simulink model "CryoDetHcd"  (R2016b)
settings: Solver=ode45  StartTime=0.0  StopTime=1e-3  RelTol=1e-3
PreLoadFcn:
  | setup_hcd
values from neighbouring files (symbols this model uses):
  A = sqrt(0.5*erfc(x))    [setup_hcd.m]
  etaRomData = zeros(1,128)    [setup_hcd.m]
  Fadc = 614e6    (= 614000000)    [setup_hcd.m]
  freqRomData = zeros(1,128)    [setup_hcd.m]
  freqRomData1 = zeros(1,128)    [setup_hcd.m]
  freqRomData2 = zeros(1,128)    [setup_hcd.m]
  freqRomData3 = zeros(1,128)    [setup_hcd.m]
undefined symbols (not defined in the file or in its folder): AXI4, B, C, D, j, Lite
libraries: xbsIndex_r4 x2151, CryoDetLibCMB x28, hdlsllib x8, dspsigops x2, simulink x1
(part 4 of 17)

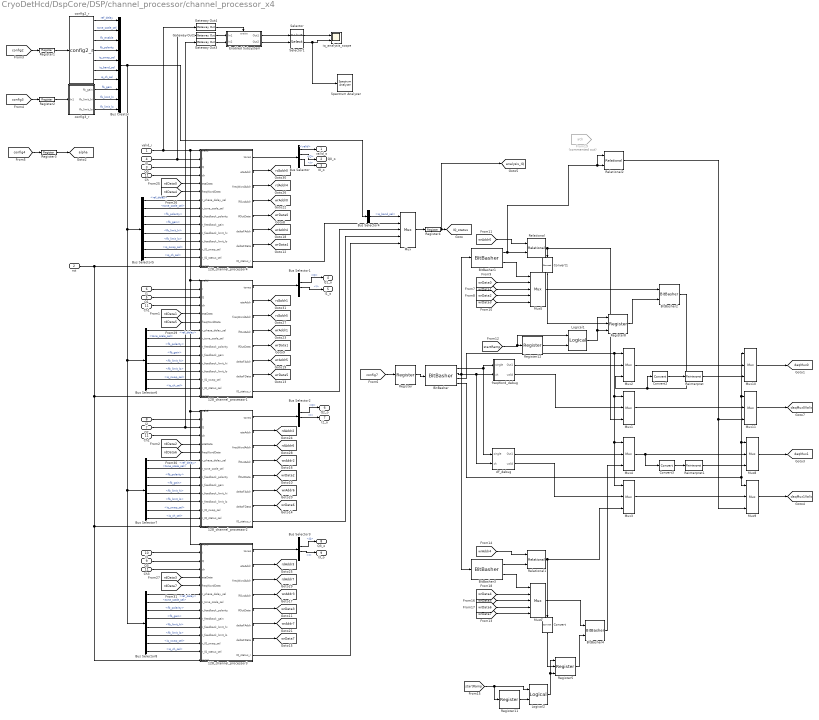
== system CryoDetHcd/DspCore/DSP/channel_processor/channel_processor_x4 ==
  valid_i : Inport
  rst : Inport  Port=2
  Q0 : Inport  Port=3
  I0 : Inport  Port=4
  Q1 : Inport  Port=5
  I1 : Inport  Port=6
  Q2 : Inport  Port=7
  I2 : Inport  Port=8
  Q3 : Inport  Port=9
  I3 : Inport  Port=10
  Ch : Inport  Port=11
  128_channel_processor1 : Subsystem  AncestorBlock=CryoDetLibCMB/128_channel_processor
  128_channel_processor2 : Subsystem  AncestorBlock=CryoDetLibCMB/128_channel_processor
  128_channel_processor3 : Subsystem  AncestorBlock=CryoDetLibCMB/128_channel_processor
  128_channel_processor4 : Subsystem  AncestorBlock=CryoDetLibCMB/128_channel_processor
  BitBasher : xbsIndex_r4/BitBasher  bitexpr=|  display_expr=off  sr_1=single_channel  arith_type1=Unsigned  bin_pt1=0  sr_2=channel_select  arith_type2=Unsigned  bin_pt2=0  sr_3=mode2  arith_type3=Unsigned  bin_pt3=0  sr_4=mode3  arith_type4=Unsigned  bin_pt4=0  dbl_ovrd=off  block_type=bitbasher
      | single_channel = {in[0]}
      | channel_select = {in[9:1]}
      | mode2 = {in[10]}
      | mode3 = {in[11]}
  BitBasher1 : xbsIndex_r4/BitBasher  bitexpr=|  display_expr=off  sr_1=ch  arith_type1=Unsigned  bin_pt1=0  sr_2=stream  arith_type2=Unsigned  bin_pt2=0  sr_3=mode2  arith_type3=Unsigned  bin_pt3=0  sr_4=4  arith_type4=Unsigned  bin_pt4=0  dbl_ovrd=off  block_type=bitbasher
      | ch = {in[6:0]}
      | stream = {in[8:7]}
  BitBasher2 : xbsIndex_r4/BitBasher  bitexpr=out = {ramp, 7'b0, in[23:0]}  display_expr=off  sr_1=out  arith_type1=Unsigned  bin_pt1=0  sr_2=channel_select  arith_type2=Unsigned  bin_pt2=0  sr_3=mode2  arith_type3=Unsigned  bin_pt3=0  sr_4=4  arith_type4=Unsigned  bin_pt4=0  dbl_ovrd=off  block_type=bitbasher
  BitBasher3 : xbsIndex_r4/BitBasher  bitexpr=|  display_expr=off  sr_1=ch  arith_type1=Unsigned  bin_pt1=0  sr_2=stream  arith_type2=Unsigned  bin_pt2=0  sr_3=mode2  arith_type3=Unsigned  bin_pt3=0  sr_4=4  arith_type4=Unsigned  bin_pt4=0  dbl_ovrd=off  block_type=bitbasher
      | ch = {in[6:0]}
      | stream = {in[8:7]}
  BitBasher4 : xbsIndex_r4/BitBasher  bitexpr=out = {ramp, 7'b0, in[23:0]}  display_expr=off  sr_1=out  arith_type1=Unsigned  bin_pt1=0  sr_2=channel_select  arith_type2=Unsigned  bin_pt2=0  sr_3=mode2  arith_type3=Unsigned  bin_pt3=0  sr_4=4  arith_type4=Unsigned  bin_pt4=0  dbl_ovrd=off  block_type=bitbasher
  Bus Creator : BusCreator  Inputs=10
  Bus Selector{,1..3} (4 alike) : BusSelector  OutputSignals=valid,Q,I,ch
  Bus Selector4 : BusSelector  OutputSignals=iq_band_sel
  Bus Selector{5..8} (4 alike) : BusSelector  OutputSignals=ref_delay,tone_scale_sel,fb_polarity,fb_gain,fb_limit_hi,fb_limit_lo,iq_swap_sel,iq_ch_sel
  Ch1 : InportShadow  Port=11
  Ch2 : InportShadow  Port=11
  Ch3 : InportShadow  Port=11
  Convert : xbsIndex_r4/Convert  gui_display_data_type=Boolean  arith_type=Boolean  n_bits=16  bin_pt=14  float_type=Single  exp_bits=8  fraction_bits=24  quantization=Truncate  overflow=Wrap  en=off  latency=0  pipeline=off  dbl_ovrd=off  block_type=convert
  Convert1 : xbsIndex_r4/Convert  gui_display_data_type=Boolean  arith_type=Boolean  n_bits=16  bin_pt=14  float_type=Single  exp_bits=8  fraction_bits=24  quantization=Truncate  overflow=Wrap  en=off  latency=0  pipeline=off  dbl_ovrd=off  block_type=convert
  Convert2 : xbsIndex_r4/Convert  gui_display_data_type=Fixed-point  arith_type="Signed  (2's comp)"  n_bits=32  bin_pt=32  float_type=Single  exp_bits=8  fraction_bits=24  quantization=Truncate  overflow=Wrap  en=off  latency=1  pipeline=off  dbl_ovrd=off  block_type=convert
  Convert3 : xbsIndex_r4/Convert  gui_display_data_type=Fixed-point  arith_type="Signed  (2's comp)"  n_bits=32  bin_pt=32  float_type=Single  exp_bits=8  fraction_bits=24  quantization=Truncate  overflow=Wrap  en=off  latency=1  pipeline=off  dbl_ovrd=off  block_type=convert
  Enabled Subsystem : Subsystem  TreatAsAtomicUnit=on
  From19 : From  Commented=on  GotoTag=aCh
  Gateway Out1 : xbsIndex_r4/Gateway Out  inherit_from_input=on  hdl_port=off  rows=1  columns=1  UseAsDAC=off  DACChannel='1'  interface=None  automatic_assignment=on  address_offset=hex2dec('00')  intf_name=''  intf_description=''  timing_constraint=None  locs_specified=off  LOCs={}  io_standard={}  block_type=gatewayout
  Gateway Out3 : xbsIndex_r4/Gateway Out  inherit_from_input=on  hdl_port=off  rows=1  columns=1  UseAsDAC=off  DACChannel='1'  interface=None  automatic_assignment=on  address_offset=hex2dec('00')  intf_name=''  intf_description=''  timing_constraint=None  locs_specified=off  LOCs={}  io_standard={}  block_type=gatewayout
  Gateway Out4 : xbsIndex_r4/Gateway Out  inherit_from_input=on  hdl_port=off  rows=1  columns=1  UseAsDAC=off  DACChannel='1'  interface=None  automatic_assignment=on  address_offset=hex2dec('00')  intf_name=''  intf_description=''  timing_constraint=None  locs_specified=off  LOCs={}  io_standard={}  block_type=gatewayout
  Logical1 : xbsIndex_r4/Logical  logical_function=OR  inputs=2  en=off  latency=0  precision=User Defined  arith_type=Boolean  n_bits=16  bin_pt=0  align_bp=on  dbl_ovrd=off  block_type=logical
  Logical2 : xbsIndex_r4/Logical  logical_function=OR  inputs=2  en=off  latency=0  precision=User Defined  arith_type=Boolean  n_bits=16  bin_pt=0  align_bp=on  dbl_ovrd=off  block_type=logical
  Mux : xbsIndex_r4/Mux  inputs=4  en=off  latency=1  precision=Full  arith_type=Unsigned  n_bits=16  bin_pt=14  quantization=Truncate  overflow=Wrap  dbl_ovrd=off  block_type=mux
  Mux{1..4,8..11} (8 alike) : xbsIndex_r4/Mux  inputs=2  en=off  latency=1  precision=Full  arith_type=Unsigned  n_bits=16  bin_pt=14  quantization=Truncate  overflow=Wrap  dbl_ovrd=off  block_type=mux
  Mux5 : xbsIndex_r4/Mux  inputs=4  en=off  latency=1  precision=Full  arith_type=Unsigned  n_bits=16  bin_pt=14  quantization=Truncate  overflow=Wrap  dbl_ovrd=off  block_type=mux
  Mux6 : xbsIndex_r4/Mux  inputs=4  en=off  latency=1  precision=Full  arith_type=Unsigned  n_bits=16  bin_pt=14  quantization=Truncate  overflow=Wrap  dbl_ovrd=off  block_type=mux
  Register{,1..4,11..12} (7 alike) : xbsIndex_r4/Register  init=0  rst=off  en=off  dbl_ovrd=off  block_type=register
  Register5 : xbsIndex_r4/Register  init=0  rst=on  en=on  dbl_ovrd=off  block_type=register
  Register8 : xbsIndex_r4/Register  init=0  rst=on  en=on  dbl_ovrd=off  block_type=register
  Reinterpret : xbsIndex_r4/Reinterpret  force_arith_type=on  arith_type=Unsigned  force_bin_pt=on  bin_pt=0  block_type=reinterpret
  Reinterpret1 : xbsIndex_r4/Reinterpret  force_arith_type=on  arith_type=Unsigned  force_bin_pt=on  bin_pt=0  block_type=reinterpret
  Relational : xbsIndex_r4/Relational  mode=a=b  op_type=Ufix  en=off  latency=1  dbl_ovrd=off  block_type=relational
  Relational1 : xbsIndex_r4/Relational  mode=a=b  op_type=Ufix  en=off  latency=1  dbl_ovrd=off  block_type=relational
  Relational2 : xbsIndex_r4/Relational  mode=a=b  op_type=Ufix  en=off  latency=1  dbl_ovrd=off  block_type=relational
  Selector : Selector  InputPortWidth=8  IndexOptions=Index vector (dialog)  Indices=[1]  OutputSizes=1
  Selector1 : Selector  InputPortWidth=8  IndexOptions=Index vector (dialog)  Indices=[1]  OutputSizes=1
  Spectrum Analyzer : SpectrumAnalyzer
  config2_r : CryoDetLibCMB/config2_r
  config3_r : Subsystem  AncestorBlock=CryoDetLibCMB/config3_r
  dF_debug : Subsystem
  freqWord_debug : Subsystem
  iq_analysis_scope : Scope  NumInputPorts=2
  valid_o : Outport
  Q0_o : Outport  Port=2
  I0_o : Outport  Port=3
  Q1_o : Outport  Port=4
  I1_o : Outport  Port=5
  Q2_o : Outport  Port=6
  I2_o : Outport  Port=7
  Q3_o : Outport  Port=8
  I3_o : Outport  Port=9
  tag scope: IQ_status=global, alpha=global, analysis_IQ=global, daqMux0=global, daqMux0Valid=global, daqMux1=global, daqMux1Valid=global, rdAddr0=global, rdAddr1=global, rdAddr2=global, rdAddr3=global, rdAddr4=global, rdAddr5=global, rdAddr6=global, rdAddr7=global, wrAddr0=global, wrAddr1=global, wrAddr2=global, wrAddr3=global, wrAddr4=global, wrAddr5=global, wrAddr6=global, wrAddr7=global, wrData0=global, wrData1=global, wrData2=global, wrData3=global, wrData4=global, wrData5=global, wrData6=global, wrData7=global
  wires:
  128_channel_processor3/8(IQ_status_r) -> Mux/5
  128_channel_processor2/8(IQ_status_r) -> Mux/4
  128_channel_processor1/8(IQ_status_r) -> Mux/3
  128_channel_processor4/8(IQ_status_r) -> Mux/2
  Register4/1 -> [analysis_IQ], [IQ_status]
  Mux/1 -> Register4/1
  Bus Selector/1 -> valid_o/1  "<valid>"
  [rdData3] -> 128_channel_processor3/5(etaData)
  [rdData7] -> 128_channel_processor3/6(freqWordData)
  [rdData6] -> 128_channel_processor2/6(freqWordData)
  [rdData2] -> 128_channel_processor2/5(etaData)
  [rdData5] -> 128_channel_processor1/6(freqWordData)
  [rdData1] -> 128_channel_processor1/5(etaData)
  128_channel_processor2/2(etaAddr) -> [rdAddr2]
  128_channel_processor2/3(freqWordAddr) -> [rdAddr6]
  128_channel_processor3/2(etaAddr) -> [rdAddr3]
  128_channel_processor3/3(freqWordAddr) -> [rdAddr7]
  128_channel_processor1/2(etaAddr) -> [rdAddr1]
  128_channel_processor1/3(freqWordAddr) -> [rdAddr5]
  128_channel_processor3/7(deltaFData) -> [wrData7]
  128_channel_processor3/6(deltaFAddr) -> [wrAddr7]
  128_channel_processor3/5(lfOutData) -> [wrData3]
  128_channel_processor3/4(lfOutAddr) -> [wrAddr3]
  128_channel_processor2/7(deltaFData) -> [wrData6]
  128_channel_processor2/6(deltaFAddr) -> [wrAddr6]
  128_channel_processor2/5(lfOutData) -> [wrData2]
  128_channel_processor2/4(lfOutAddr) -> [wrAddr2]
  128_channel_processor1/4(lfOutAddr) -> [wrAddr1]
  128_channel_processor1/5(lfOutData) -> [wrData1]
  128_channel_processor1/6(deltaFAddr) -> [wrAddr5]
  128_channel_processor1/7(deltaFData) -> [wrData5]
  Q1/1 -> 128_channel_processor1/3(Q)
  I1/1 -> 128_channel_processor1/2(I)
  I2/1 -> 128_channel_processor2/2(I)
  I3/1 -> 128_channel_processor3/2(I)
  Q3/1 -> 128_channel_processor3/3(Q)
  Bus Selector3/3 -> I3_o/1  "<I>"
  Bus Selector3/2 -> Q3_o/1  "<Q>"
  Bus Selector2/3 -> I2_o/1  "<I>"
  Bus Selector2/2 -> Q2_o/1  "<Q>"
  Bus Selector1/3 -> I1_o/1  "<I>"
  Bus Selector1/2 -> Q1_o/1  "<Q>"
  128_channel_processor3/1(tones) -> Bus Selector3/1
  128_channel_processor2/1(tones) -> Bus Selector2/1
  128_channel_processor1/1(tones) -> Bus Selector1/1
  Bus Selector/3 -> I0_o/1  "<I>"
  Bus Selector/2 -> Q0_o/1  "<Q>"
  128_channel_processor4/1(tones) -> Bus Selector/1
  Ch/1 -> 128_channel_processor4/4(ch)
  [rdData4] -> 128_channel_processor4/6(freqWordData)
  [rdData0] -> 128_channel_processor4/5(etaData)
  128_channel_processor4/7(deltaFData) -> [wrData4]
  128_channel_processor4/5(lfOutData) -> [wrData0]
  128_channel_processor4/4(lfOutAddr) -> [wrAddr0]
  128_channel_processor4/6(deltaFAddr) -> [wrAddr4]
  128_channel_processor4/2(etaAddr) -> [rdAddr0]
  128_channel_processor4/3(freqWordAddr) -> [rdAddr4]
  [config2] -> Register1/1
  [config3] -> Register2/1
  Register2/1 -> config3_r/1(In1)
  Register1/1 -> config2_r/1
  config2_r/5 -> Bus Creator/5  "iq_swap_sel"
  config2_r/7 -> Bus Creator/7  "iq_ch_sel"
  config2_r/6 -> Bus Creator/6  "iq_band_sel"
  config2_r/1 -> Bus Creator/1  "ref_delay"
  config2_r/2 -> Bus Creator/2  "tone_scale_sel"
  config2_r/3 -> Bus Creator/3  "fb_enable"
  config2_r/4 -> Bus Creator/4  "fb_polarity"
  config3_r/1(fb_gain) -> Bus Creator/8  "fb_gain"
  config3_r/2(fb_limit_hi) -> Bus Creator/9  "fb_limit_hi"
  Bus Selector4/1 -> Mux/1  "<iq_band_sel>"
  Bus Creator/1 -> Bus Selector4/1, Bus Selector6/1, Bus Selector8/1, Bus Selector7/1, Bus Selector5/1
  Ch1/1 -> 128_channel_processor1/4(ch)
  Ch2/1 -> 128_channel_processor2/4(ch)
  Ch3/1 -> 128_channel_processor3/4(ch)
  config3_r/3(fb_limit_lo) -> Bus Creator/10  "fb_limit_lo"
  Bus Selector5/2 -> 128_channel_processor4/8(r_tone_scale_sel)  "<tone_scale_sel>"
  Bus Selector5/3 -> 128_channel_processor4/9(r_feedback_polarity)  "<fb_polarity>"
  Bus Selector5/1 -> 128_channel_processor4/7(r_phase_delay_sel)  "<ref_delay>"
  Bus Selector5/4 -> 128_channel_processor4/10(r_feedback_gain)  "<fb_gain>"
  Bus Selector5/5 -> 128_channel_processor4/11(r_feedback_limit_hi)  "<fb_limit_hi>"
  Bus Selector5/6 -> 128_channel_processor4/12(r_feedback_limit_lo)  "<fb_limit_lo>"
  Bus Selector5/7 -> 128_channel_processor4/13(r_IQ_swap_sel)  "<iq_swap_sel>"
  Bus Selector5/8 -> 128_channel_processor4/14(r_IQ_status_sel)  "<iq_ch_sel>"
  Bus Selector6/7 -> 128_channel_processor1/13(r_IQ_swap_sel)  "<iq_swap_sel>"
  Bus Selector6/8 -> 128_channel_processor1/14(r_IQ_status_sel)  "<iq_ch_sel>"
  Bus Selector6/1 -> 128_channel_processor1/7(r_phase_delay_sel)  "<ref_delay>"
  Bus Selector6/4 -> 128_channel_processor1/10(r_feedback_gain)  "<fb_gain>"
  Bus Selector6/5 -> 128_channel_processor1/11(r_feedback_limit_hi)  "<fb_limit_hi>"
  Bus Selector6/6 -> 128_channel_processor1/12(r_feedback_limit_lo)  "<fb_limit_lo>"
  Bus Selector6/3 -> 128_channel_processor1/9(r_feedback_polarity)  "<fb_polarity>"
  Bus Selector6/2 -> 128_channel_processor1/8(r_tone_scale_sel)  "<tone_scale_sel>"
  Bus Selector7/6 -> 128_channel_processor2/12(r_feedback_limit_lo)  "<fb_limit_lo>"
  Bus Selector7/1 -> 128_channel_processor2/7(r_phase_delay_sel)  "<ref_delay>"
  Bus Selector7/5 -> 128_channel_processor2/11(r_feedback_limit_hi)  "<fb_limit_hi>"
  Bus Selector7/2 -> 128_channel_processor2/8(r_tone_scale_sel)  "<tone_scale_sel>"
  Bus Selector7/7 -> 128_channel_processor2/13(r_IQ_swap_sel)  "<iq_swap_sel>"
  Bus Selector7/3 -> 128_channel_processor2/9(r_feedback_polarity)  "<fb_polarity>"
  Bus Selector7/4 -> 128_channel_processor2/10(r_feedback_gain)  "<fb_gain>"
  Bus Selector7/8 -> 128_channel_processor2/14(r_IQ_status_sel)  "<iq_ch_sel>"
  rst/1 -> 128_channel_processor4/15(reset), 128_channel_processor1/15(reset), 128_channel_processor3/15(reset), 128_channel_processor2/15(reset)
  Bus Selector8/8 -> 128_channel_processor3/14(r_IQ_status_sel)  "<iq_ch_sel>"
  Bus Selector8/4 -> 128_channel_processor3/10(r_feedback_gain)  "<fb_gain>"
  Bus Selector8/2 -> 128_channel_processor3/8(r_tone_scale_sel)  "<tone_scale_sel>"
  Bus Selector8/3 -> 128_channel_processor3/9(r_feedback_polarity)  "<fb_polarity>"
  Bus Selector8/1 -> 128_channel_processor3/7(r_phase_delay_sel)  "<ref_delay>"
  Bus Selector8/5 -> 128_channel_processor3/11(r_feedback_limit_hi)  "<fb_limit_hi>"
  Bus Selector8/6 -> 128_channel_processor3/12(r_feedback_limit_lo)  "<fb_limit_lo>"
  Bus Selector8/7 -> 128_channel_processor3/13(r_IQ_swap_sel)  "<iq_swap_sel>"
  [config4] -> Register3/1
  Register3/1 -> [alpha]
  I0/1 -> Gateway Out1/1, 128_channel_processor4/2(I)
  Q0/1 -> 128_channel_processor4/3(Q)
  valid_i/1 -> Gateway Out4/1, 128_channel_processor4/1(valid), 128_channel_processor1/1(valid), 128_channel_processor3/1(valid), 128_channel_processor2/1(valid)
  Enabled Subsystem/2(Out2) -> Selector1/1
  Enabled Subsystem/1(Out1) -> Selector/1
  Selector1/1 -> Spectrum Analyzer/1, iq_analysis_scope/2
  Selector/1 -> iq_analysis_scope/1
  Gateway Out1/1 -> Enabled Subsystem/1(In1)
  Gateway Out3/1 -> Enabled Subsystem/2(In2)
  Gateway Out4/1 -> Enabled Subsystem/Enable
  Q2/1 -> 128_channel_processor2/3(Q), Gateway Out3/1
  [config7] -> Register/1
  Register/1 -> BitBasher/1
  BitBasher/1 -> freqWord_debug/1(single), dF_debug/1(single)
  BitBasher/2 -> BitBasher3/1, BitBasher1/1, dF_debug/2(ch), freqWord_debug/2(ch)
  freqWord_debug/1(Out1) -> Mux2/2
  freqWord_debug/2(valid) -> Mux1/2
  BitBasher/3 -> Mux4/1, Mux3/1, Mux1/1, Mux2/1
  dF_debug/1(Out1) -> Mux4/2
  dF_debug/2(valid) -> Mux3/2
  BitBasher1/2 -> Mux5/1
  [wrData0] -> Mux5/2
  [wrData1] -> Mux5/3
  [wrData3] -> Mux5/5
  [wrData2] -> Mux5/4
  [wrAddr0] -> Relational/1
  BitBasher3/2 -> Mux6/1
  [wrData4] -> Mux6/2
  [wrData5] -> Mux6/3
  [wrData7] -> Mux6/5
  [wrData6] -> Mux6/4
  BitBasher3/1 -> Relational1/2
  [wrAddr4] -> Relational1/1
  BitBasher4/1 -> Mux4/3
  Mux6/1 -> BitBasher4/1
  Relational1/1 -> Mux3/3, Convert/1
  Mux5/1 -> BitBasher2/1
  Relational/1 -> Mux1/3, Convert1/1
  [startRamp] -> Logical1/1, Register12/1
  [startRamp] -> Register11/1, Logical2/1
  Convert/1 -> Register5/2
  Convert1/1 -> Register8/2
  Register8/1 -> BitBasher2/2
  Register12/1 -> Logical1/2
  Logical1/1 -> Register8/1, Register8/3
  Register11/1 -> Logical2/2
  Logical2/1 -> Register5/1, Register5/3
  Register5/1 -> BitBasher4/2
  BitBasher2/1 -> Convert2/1, Mux2/3
  Mux4/1 -> Convert3/1, Mux8/2
  Mux8/1 -> [daqMux1]
  Mux3/1 -> Mux9/2
  Mux9/1 -> [daqMux1Valid]
  Mux1/1 -> Mux11/2
  Mux11/1 -> [daqMux0Valid]
  Mux2/1 -> Mux10/2
  Mux10/1 -> [daqMux0]
  Convert3/1 -> Reinterpret1/1
  Convert2/1 -> Reinterpret/1
  Relational2/1 -> Mux9/3, Mux11/3
  BitBasher/4 -> Mux9/1, Mux11/1, Mux10/1, Mux8/1
  Reinterpret/1 -> Mux10/3
  Reinterpret1/1 -> Mux8/3
  BitBasher1/1 -> Relational2/1, Relational2/2, Relational/2

== system CryoDetHcd/DspCore/DSP/Synthesis_pipelined/Synthesis/Combine ==
  valid : Inport
  im0 : Inport  Port=2
  re0 : Inport  Port=3
  im1 : Inport  Port=4
  re1 : Inport  Port=5
  Add2 : Sum
  AddSub{,1..3} (4 alike) : xbsIndex_r4/AddSub  mode=Subtraction  use_carryin=off  use_carryout=off  en=off  latency=2  precision=User Defined  arith_type="Signed  (2's comp)"  n_bits=16  bin_pt=15  quantization=Truncate  overflow=Saturate  use_behavioral_HDL=on  hw_selection=Fabric  pipelined=off  dbl_ovrd=off  block_type=addsub
  BitBasher1 : xbsIndex_r4/BitBasher  bitexpr=|  display_expr=off  sr_1=hi  arith_type1="Signed  (2's comp)"  bin_pt1=15  sr_2=lo  arith_type2="Signed  (2's comp)"  bin_pt2=15  sr_3=hi  arith_type3=Unsigned  bin_pt3=0  sr_4=4  arith_type4=Unsigned  bin_pt4=0  dbl_ovrd=off  block_type=bitbasher
      | hi = {in[31:16]}
      | lo = {in[15:0]}
  BitBasher2 : xbsIndex_r4/BitBasher  bitexpr=|  display_expr=off  sr_1=hi  arith_type1="Signed  (2's comp)"  bin_pt1=15  sr_2=lo  arith_type2="Signed  (2's comp)"  bin_pt2=15  sr_3=hi  arith_type3=Unsigned  bin_pt3=0  sr_4=4  arith_type4=Unsigned  bin_pt4=0  dbl_ovrd=off  block_type=bitbasher
      | hi = {in[31:16]}
      | lo = {in[15:0]}
  BitBasher3 : xbsIndex_r4/BitBasher  bitexpr=|  display_expr=off  sr_1=hi  arith_type1="Signed  (2's comp)"  bin_pt1=15  sr_2=lo  arith_type2="Signed  (2's comp)"  bin_pt2=15  sr_3=hi  arith_type3=Unsigned  bin_pt3=0  sr_4=4  arith_type4=Unsigned  bin_pt4=0  dbl_ovrd=off  block_type=bitbasher
      | hi = {in[31:16]}
      | lo = {in[15:0]}
  BitBasher4 : xbsIndex_r4/BitBasher  bitexpr=|  display_expr=off  sr_1=hi  arith_type1="Signed  (2's comp)"  bin_pt1=15  sr_2=lo  arith_type2="Signed  (2's comp)"  bin_pt2=15  sr_3=hi  arith_type3=Unsigned  bin_pt3=0  sr_4=4  arith_type4=Unsigned  bin_pt4=0  dbl_ovrd=off  block_type=bitbasher
      | hi = {in[31:16]}
      | lo = {in[15:0]}
  BitBasher5 : xbsIndex_r4/BitBasher  bitexpr=out = {hi, lo}  display_expr=off  sr_1=out  arith_type1=Unsigned  bin_pt1=0  sr_2=hi  arith_type2="Signed  (2's comp)"  bin_pt2=15  sr_3=hi  arith_type3=Unsigned  bin_pt3=0  sr_4=4  arith_type4=Unsigned  bin_pt4=0  dbl_ovrd=off  block_type=bitbasher
  BitBasher6 : xbsIndex_r4/BitBasher  bitexpr=out = {hi, lo}  display_expr=off  sr_1=out  arith_type1=Unsigned  bin_pt1=0  sr_2=hi  arith_type2="Signed  (2's comp)"  bin_pt2=15  sr_3=hi  arith_type3=Unsigned  bin_pt3=0  sr_4=4  arith_type4=Unsigned  bin_pt4=0  dbl_ovrd=off  block_type=bitbasher
  Dac{1..4} (4 alike) : xbsIndex_r4/Gateway Out  inherit_from_input=off  hdl_port=off  rows=1  columns=1  UseAsDAC=off  DACChannel='1'  interface=None  automatic_assignment=on  address_offset=hex2dec('00')  intf_name=''  intf_description=''  timing_constraint=None  locs_specified=off  LOCs={}  io_standard={}  block_type=gatewayout
  Delay : xbsIndex_r4/Delay  rst=off  infoeditControl=Selection of Reset will increase slice count due to use of real FFs and instead of SRLs  en=off  latency=4  reg_retiming=on  dbl_ovrd=off  block_type=delay
  Delay11 : Delay  DelayLength=1
  Real-Imag to Complex2 : RealImagToComplex
  Real-Imag to Complex3 : RealImagToComplex
  Register{,1..11} (12 alike) : xbsIndex_r4/Register  init=0  rst=off  en=off  dbl_ovrd=off  block_type=register
  Scale{,1..3} (4 alike) : xbsIndex_r4/Scale  scale_factor=15  dbl_ovrd=off  block_type=scale
  Scope : Scope
  Spectrum Analyzer : SpectrumAnalyzer
  Upsample : dspsigops/Upsample  N=2  phase=0  RateOptions=Allow multirate processing  ic=0  mode=Unused parameter value
  Upsample4 : dspsigops/Upsample  N=2  phase=0  RateOptions=Allow multirate processing  ic=0  mode=Unused parameter value
  valid0 : Outport
  im_o : Outport  Port=2
  re_o : Outport  Port=3
  wires:
  Register11/1 -> AddSub3/2
  Register10/1 -> AddSub3/1
  Register9/1 -> AddSub2/2
  Register8/1 -> AddSub2/1
  Register7/1 -> AddSub1/2
  Register6/1 -> AddSub1/1
  Register5/1 -> AddSub/2
  Register4/1 -> AddSub/1
  BitBasher5/1 -> im_o/1
  BitBasher6/1 -> re_o/1
  AddSub3/1 -> Register3/1
  AddSub2/1 -> Register2/1
  AddSub1/1 -> Register1/1
  AddSub/1 -> Register/1
  Delay/1 -> valid0/1
  BitBasher2/2 -> Register11/1
  BitBasher3/2 -> Register10/1
  BitBasher2/1 -> Register9/1
  BitBasher3/1 -> Register8/1
  re0/1 -> BitBasher3/1
  re1/1 -> BitBasher2/1
  BitBasher1/2 -> Register7/1
  BitBasher4/2 -> Register6/1
  BitBasher1/1 -> Register5/1
  BitBasher4/1 -> Register4/1
  valid/1 -> Delay/1
  im0/1 -> BitBasher4/1
  im1/1 -> BitBasher1/1
  Real-Imag to Complex3/1 -> Upsample4/1
  Dac4/1 -> Real-Imag to Complex2/2
  Dac1/1 -> Real-Imag to Complex3/2
  Add2/1 -> Scope/1, Spectrum Analyzer/1
  Dac2/1 -> Real-Imag to Complex3/1
  Delay11/1 -> Add2/2
  Upsample4/1 -> Delay11/1
  Dac3/1 -> Real-Imag to Complex2/1
  Register1/1 -> BitBasher5/1, Scale3/1
  Register3/1 -> BitBasher6/1, Scale2/1
  Register2/1 -> Scale/1, BitBasher6/2
  Register/1 -> BitBasher5/2, Scale1/1
  Upsample/1 -> Add2/1
  Scale/1 -> Dac3/1
  Scale1/1 -> Dac4/1
  Real-Imag to Complex2/1 -> Upsample/1
  Scale2/1 -> Dac2/1
  Scale3/1 -> Dac1/1

== system CryoDetHcd/DspCore/DSP/Synthesis_pipelined/Synthesis/Post_synthesis0 ==
  valid : Inport
  im : Inport  Port=2
  re : Inport  Port=3
  Delay : xbsIndex_r4/Delay  rst=off  infoeditControl=Selection of Reset will increase slice count due to use of real FFs and instead of SRLs  en=off  latency=9  reg_retiming=on  dbl_ovrd=off  block_type=delay
  Delay1 : xbsIndex_r4/Delay  rst=off  infoeditControl=Selection of Reset will increase slice count due to use of real FFs and instead of SRLs  en=off  latency=9  reg_retiming=on  dbl_ovrd=off  block_type=delay
  Delay2 : xbsIndex_r4/Delay  rst=off  infoeditControl=Selection of Reset will increase slice count due to use of real FFs and instead of SRLs  en=off  latency=9  reg_retiming=on  dbl_ovrd=off  block_type=delay
  valid0 : Outport
  im0 : Outport  Port=2
  reo : Outport  Port=3
  wires:
  Delay2/1 -> reo/1
  Delay1/1 -> im0/1
  Delay/1 -> valid0/1
  re/1 -> Delay2/1
  im/1 -> Delay1/1
  valid/1 -> Delay/1

== system CryoDetHcd/DspCore/DSP/Synthesis_pipelined/Synthesis/Post_sytnehsis1 ==
  valid : Inport
  im : Inport  Port=2
  re : Inport  Port=3
  BitBasher1 : xbsIndex_r4/BitBasher  bitexpr=|  display_expr=off  sr_1=hi  arith_type1="Signed  (2's comp)"  bin_pt1=15  sr_2=lo  arith_type2="Signed  (2's comp)"  bin_pt2=15  sr_3=hi  arith_type3=Unsigned  bin_pt3=0  sr_4=4  arith_type4=Unsigned  bin_pt4=0  dbl_ovrd=off  block_type=bitbasher
      | hi = {in[31:16]}
      | lo = {in[15:0]}
  BitBasher2 : xbsIndex_r4/BitBasher  bitexpr=out = {hi, lo}  display_expr=off  sr_1=out  arith_type1=Unsigned  bin_pt1=0  sr_2=hi  arith_type2="Signed  (2's comp)"  bin_pt2=15  sr_3=hi  arith_type3=Unsigned  bin_pt3=0  sr_4=4  arith_type4=Unsigned  bin_pt4=0  dbl_ovrd=off  block_type=bitbasher
  BitBasher3 : xbsIndex_r4/BitBasher  bitexpr=out = {hi, lo}  display_expr=off  sr_1=out  arith_type1=Unsigned  bin_pt1=0  sr_2=hi  arith_type2="Signed  (2's comp)"  bin_pt2=15  sr_3=hi  arith_type3=Unsigned  bin_pt3=0  sr_4=4  arith_type4=Unsigned  bin_pt4=0  dbl_ovrd=off  block_type=bitbasher
  BitBasher4 : xbsIndex_r4/BitBasher  bitexpr=|  display_expr=off  sr_1=hi  arith_type1="Signed  (2's comp)"  bin_pt1=15  sr_2=lo  arith_type2="Signed  (2's comp)"  bin_pt2=15  sr_3=hi  arith_type3=Unsigned  bin_pt3=0  sr_4=4  arith_type4=Unsigned  bin_pt4=0  dbl_ovrd=off  block_type=bitbasher
      | hi = {in[31:16]}
      | lo = {in[15:0]}
  "Complex Multiplier 6.0 " : xbsIndex_r4/Complex Multiplier 6.0   hasatlast=off  hasatuser=off  atuserwidth=1  hasbtlast=off  hasbtuser=off  btuserwidth=1  multtype=Use_Mults  optimizegoal=Resources  flowcontrol=NonBlocking  outputwidth=19  roundmode=Truncate  hasctrltlast=off  hasctrltuser=off  ctrltuserwidth=1  outtlastbehv=Null  latencyconfig=Automatic  minimumlatency=37  aclken=off  aresetn=off  trim_axipin_name=on  simulation_type=hybrid_sim  simulation_model=sysgen:cmpy_v6_0  data_path_portlist={ 's_axis_a_tdata_real', 's_axis_a_tdata_imag', 's_axis_b_tdata_real', 's_axis_b_tdata_imag', 's_axis_ctrl_tdata_rounding_bit', 'm_axis_dout_tdata_real', 'm_axis_dout_tdata_imag' }  aportwidth=63  bportwidth=63  ip_name=Complex Multiplier  ip_version=6.0  dsptool_ready=true  ipcore_usecache=true  ipcore_useipmodelcache=true  ipcore_verbose=false  ipcore_latency_parameter='minimumlatency'  wrapper_available=true  port_translation_map={ 'aclken' => 'en', 'aresetn' => 'rst'}  block_type=cmpy_v6_0
  Complex Multiplier 6.0 1 : xbsIndex_r4/Complex Multiplier 6.0   hasatlast=off  hasatuser=off  atuserwidth=1  hasbtlast=off  hasbtuser=off  btuserwidth=1  multtype=Use_Mults  optimizegoal=Resources  flowcontrol=NonBlocking  outputwidth=19  roundmode=Truncate  hasctrltlast=off  hasctrltuser=off  ctrltuserwidth=1  outtlastbehv=Null  latencyconfig=Automatic  minimumlatency=37  aclken=off  aresetn=off  trim_axipin_name=on  simulation_type=hybrid_sim  simulation_model=sysgen:cmpy_v6_0  data_path_portlist={ 's_axis_a_tdata_real', 's_axis_a_tdata_imag', 's_axis_b_tdata_real', 's_axis_b_tdata_imag', 's_axis_ctrl_tdata_rounding_bit', 'm_axis_dout_tdata_real', 'm_axis_dout_tdata_imag' }  aportwidth=63  bportwidth=63  ip_name=Complex Multiplier  ip_version=6.0  dsptool_ready=true  ipcore_usecache=true  ipcore_useipmodelcache=true  ipcore_verbose=false  ipcore_latency_parameter='minimumlatency'  wrapper_available=true  port_translation_map={ 'aclken' => 'en', 'aresetn' => 'rst'}  block_type=cmpy_v6_0
  Convert{,1..3} (4 alike) : xbsIndex_r4/Convert  gui_display_data_type=Fixed-point  arith_type="Signed  (2's comp)"  n_bits=16  bin_pt=15  float_type=Single  exp_bits=8  fraction_bits=24  quantization=Truncate  overflow=Flag as error  en=off  latency=0  pipeline=off  dbl_ovrd=off  block_type=convert
  Counter : xbsIndex_r4/Counter  cnt_type=Free Running  cnt_to=Inf  operation=Up  start_count=2  cnt_by_val=1  arith_type=Unsigned  n_bits=4  bin_pt=0  load_pin=off  rst=on  en=on  explicit_period=on  period=2/Fadc  use_behavioral_HDL=off  implementation=Fabric  dbl_ovrd=off  block_type=counter
  Register{,1..10,44} (12 alike) : xbsIndex_r4/Register  init=0  rst=off  en=off  dbl_ovrd=off  block_type=register
  imag1 : xbsIndex_r4/ROM  depth=16  initVector=imag(exp(j*2*pi*(1:2:31)/32))  distributed_mem=Block RAM  rst=off  init_reg=0  en=off  latency=2  gui_display_data_type=Fixed-point  arith_type="Signed  (2's comp)"  n_bits=18  bin_pt=16  preci_type=Single  exp_width=8  frac_width=24  optimize=Area  use_rpm=on  dbl_ovrd=off  block_type=sprom
  imag2 : xbsIndex_r4/ROM  depth=16  initVector=imag(exp(j*2*pi*(0:2:31)/32))  distributed_mem=Block RAM  rst=off  init_reg=0  en=off  latency=2  gui_display_data_type=Fixed-point  arith_type="Signed  (2's comp)"  n_bits=18  bin_pt=16  preci_type=Single  exp_width=8  frac_width=24  optimize=Area  use_rpm=on  dbl_ovrd=off  block_type=sprom
  real1 : xbsIndex_r4/ROM  depth=16  initVector=real(exp(j*2*pi*(1:2:31)/32))  distributed_mem=Block RAM  rst=off  init_reg=0  en=off  latency=2  gui_display_data_type=Fixed-point  arith_type="Signed  (2's comp)"  n_bits=18  bin_pt=16  preci_type=Single  exp_width=8  frac_width=24  optimize=Area  use_rpm=on  dbl_ovrd=off  block_type=sprom
  real2 : xbsIndex_r4/ROM  depth=16  initVector=real(exp(j*2*pi*(0:2:31)/32))  distributed_mem=Block RAM  rst=off  init_reg=0  en=off  latency=2  gui_display_data_type=Fixed-point  arith_type="Signed  (2's comp)"  n_bits=18  bin_pt=16  preci_type=Single  exp_width=8  frac_width=24  optimize=Area  use_rpm=on  dbl_ovrd=off  block_type=sprom
  valid0 : Outport
  im0 : Outport  Port=2
  reo : Outport  Port=3
  wires:
  Register10/1 -> BitBasher1/1
  Register9/1 -> BitBasher4/1
  Register8/1 -> reo/1
  Register5/1 -> im0/1
  Register4/1 -> valid0/1
  real1/1 -> Complex Multiplier 6.0 1/6
  imag1/1 -> Complex Multiplier 6.0 1/5
  Register7/1 -> Complex Multiplier 6.0 1/3
  Register6/1 -> Complex Multiplier 6.0 1/2
  real2/1 -> "Complex Multiplier 6.0 "/6
  imag2/1 -> "Complex Multiplier 6.0 "/5
  Register3/1 -> "Complex Multiplier 6.0 "/3
  Register2/1 -> "Complex Multiplier 6.0 "/2
  Register1/1 -> "Complex Multiplier 6.0 "/1, Complex Multiplier 6.0 1/4, Complex Multiplier 6.0 1/1, "Complex Multiplier 6.0 "/4
  BitBasher4/2 -> Register6/1
  BitBasher1/2 -> Register7/1
  BitBasher1/1 -> Register3/1
  BitBasher4/1 -> Register2/1
  "Complex Multiplier 6.0 "/2 -> Convert/1
  "Complex Multiplier 6.0 "/3 -> Convert2/1
  Complex Multiplier 6.0 1/3 -> Convert3/1
  Complex Multiplier 6.0 1/2 -> Convert1/1
  Convert1/1 -> BitBasher2/2
  "Complex Multiplier 6.0 "/1 -> Register4/1
  Register/1 -> Register1/1
  Convert3/1 -> BitBasher3/2
  Convert2/1 -> BitBasher3/1
  Convert/1 -> BitBasher2/1
  BitBasher3/1 -> Register8/1
  BitBasher2/1 -> Register5/1
  Counter/1 -> real1/1, imag1/1, real2/1, imag2/1
  re/1 -> Register10/1
  im/1 -> Register9/1
  valid/1 -> Counter/2, Register/1
  [reset] -> Register44/1
  Register44/1 -> Counter/1
